simulink model "Chap6_RealBaseband"  (R2016a)
settings: Solver=VariableStepDiscrete  StartTime=0.0  StopTime=1  RelTol=1e-3
InitFcn:
  | clear
  | BitRate = 4e6;
  | SamplePerFrame = 4000;
  | SNR = 10;
  | M = 4;
  | l = log2(M);
  | 
  | % 实数通过AWGN
  | EsN0 = SNR - 10 * log10(2);
  | EbN0 = EsN0 - 10 * log10(l);
  | BER1Theory = berawgn(EbN0, 'pam', M);
  | 
  | % 复数通过AWGN
  | EsN0 = SNR;
  | EbN0 = EsN0 - 10 * log10(l);
  | BER2Theory = berawgn(EbN0, 'pam', M);
libraries: commdigbbndam3 x4, commchan3 x2, commsink2 x2, commrandsrc2 x1
settings Model: Creator=Administrator  LastModifiedBy=Administrator
settings DataIOCC: LimitDataPoints=on  SaveFormat=Array
settings DebuggingCC: SignalRangeChecking=warning  ParameterOverflowMsg=warning  ParameterPrecisionLossMsg=none  ParameterTunabilityLossMsg=none
settings HardwareCC: ProdBitPerPointer=32  ProdLargestAtomicFloat=None  ProdIntDivRoundTo=Undefined  ProdEndianess=Unspecified  ProdWordSize=32  ProdHWDeviceType=ASIC/FPGA->ASIC/FPGA  TargetHWDeviceType=Generic->Custom  ProdEqTarget=off
settings ModelReferenceCC: PropagateSignalLabelsOutOfModel=off
settings ConfigComp: CovModelRefEnable=Off

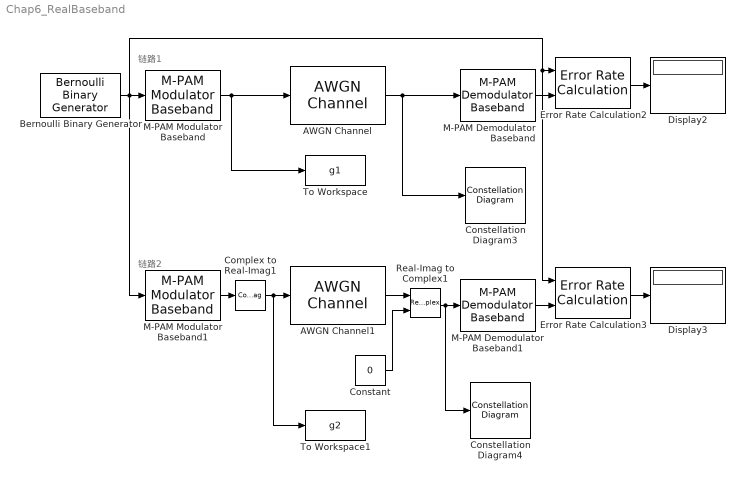
== system Chap6_RealBaseband ==
  note: 链路1
  note: 链路2
  AWGN Channel : commchan3/AWGN Channel  InputProcessing=Columns as channels (frame based)  seed=67  noiseMode="Signal to noise ratio  (SNR)"  EbNodB=10  EsNodB=10  SNRdB=SNR  bitsPerSym=4  Ps=1  Tsym=4e-6  variance=1
  AWGN Channel1 : commchan3/AWGN Channel  InputProcessing=Columns as channels (frame based)  seed=67  noiseMode="Signal to noise ratio  (SNR)"  EbNodB=10  EsNodB=10  SNRdB=SNR  bitsPerSym=4  Ps=1  Tsym=4e-6  variance=1
  Bernoulli Binary Generator : commrandsrc2/Bernoulli Binary Generator  P=0.5  seed=61  Ts=1/BitRate  frameBased=on  sampPerFrame=SamplePerFrame  orient=off  outDataType=double
  Complex to Real-Imag1 : ComplexToRealImag  Output=Real
  Constant : Constant  Value=0
  Constellation Diagram3 : ConstellationDiagram
  Constellation Diagram4 : ConstellationDiagram
  Display2 : Display
  Display3 : Display
  Error Rate Calculation2 : commsink2/Error Rate Calculation  N=0  st_delay=0  cp_mode=Entire frame  subframe=[]  PMode=Port  WsName=ErrorVec  RsMode2=off  stop=off  numErr=100  maxBits=1e6
  Error Rate Calculation3 : commsink2/Error Rate Calculation  N=0  st_delay=0  cp_mode=Entire frame  subframe=[]  PMode=Port  WsName=ErrorVec  RsMode2=off  stop=off  numErr=100  maxBits=1e6
  M-PAM Demodulator Baseband : commdigbbndam3/M-PAM Demodulator Baseband  M=4  OutType=Bit  Dec=Gray  PowType=Average Power  MinDist=2  AvgPow=1  PeakPow=1  outDtype1=Inherit via internal rule  outDtype2=Inherit via internal rule  denormFactorWordLen=16  denormFactorDataTypeStr=Inherit: Same word length as input  denormFactorLastDataTypeStr=Inherit: Same word length as input  prodOutWordLen=16  prodOutRoundingMode=Floor  prodOutOverflowMode=Wrap  prodOutOvFlMode=off  prodOutOvFlModeLastStrValue=off  sumWordLen=16
  M-PAM Demodulator Baseband1 : commdigbbndam3/M-PAM Demodulator Baseband  M=4  OutType=Bit  Dec=Gray  PowType=Average Power  MinDist=2  AvgPow=1  PeakPow=1  outDtype1=Inherit via internal rule  outDtype2=Inherit via internal rule  denormFactorWordLen=16  denormFactorDataTypeStr=Inherit: Same word length as input  denormFactorLastDataTypeStr=Inherit: Same word length as input  prodOutWordLen=16  prodOutRoundingMode=Floor  prodOutOverflowMode=Wrap  prodOutOvFlMode=off  prodOutOvFlModeLastStrValue=off  sumWordLen=16
  M-PAM Modulator Baseband : commdigbbndam3/M-PAM Modulator Baseband  M=4  InType=Bit  Enc=Gray  PowType=Average Power  MinDist=2  AvgPow=1  PeakPow=1  outDtype=double  outWordLen=16  outUDDataType=sfix(16)  outFracLenMode=Best precision  outFracLen=15  outDataTypeStr=double  outLastDataTypeStr=double
  M-PAM Modulator Baseband1 : commdigbbndam3/M-PAM Modulator Baseband  M=4  InType=Bit  Enc=Gray  PowType=Average Power  MinDist=2  AvgPow=1  PeakPow=1  outDtype=double  outWordLen=16  outUDDataType=sfix(16)  outFracLenMode=Best precision  outFracLen=15  outDataTypeStr=double  outLastDataTypeStr=double
  Real-Imag to Complex1 : RealImagToComplex
  To Workspace : ToWorkspace  VariableName=g1  SampleTime=-1
      settings: Save2DSignal=2-D array (concatenate along first dimension)
  To Workspace1 : ToWorkspace  VariableName=g2  SampleTime=-1
      settings: Save2DSignal=2-D array (concatenate along first dimension)
  wires:
  M-PAM Modulator Baseband/1 -> To Workspace/1, AWGN Channel/1
  AWGN Channel/1 -> Constellation Diagram3/1, M-PAM Demodulator Baseband/1
  Error Rate Calculation2/1 -> Display2/1
  M-PAM Demodulator Baseband/1 -> Error Rate Calculation2/2
  M-PAM Modulator Baseband1/1 -> Complex to Real-Imag1/1
  Real-Imag to Complex1/1 -> Constellation Diagram4/1, M-PAM Demodulator Baseband1/1
  Error Rate Calculation3/1 -> Display3/1
  M-PAM Demodulator Baseband1/1 -> Error Rate Calculation3/2
  Complex to Real-Imag1/1 -> To Workspace1/1, AWGN Channel1/1
  AWGN Channel1/1 -> Real-Imag to Complex1/1
  Constant/1 -> Real-Imag to Complex1/2
  Bernoulli Binary Generator/1 -> Error Rate Calculation2/1, Error Rate Calculation3/1, M-PAM Modulator Baseband/1, M-PAM Modulator Baseband1/1
